simulink model "ARS308_RX"  (R2018b)
settings: Solver=FixedStepAuto  StartTime=0.0  StopTime=inf  FixedStep=0.005  RelTol=1e-3
PostLoadFcn:
  | if any(exist('dsrtsu_mdlpostloadfcn', 'file') ~= 0), dsrtsu_mdlpostloadfcn('Execute', bdroot); end
libraries: rtican x18
(part 4 of 4)

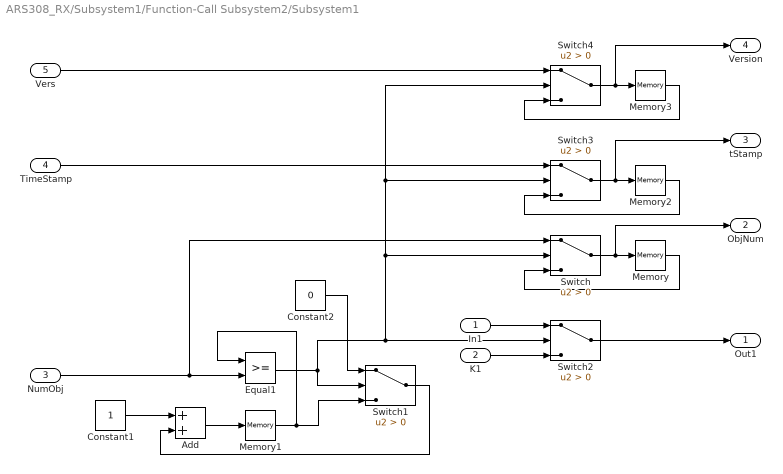
== system ARS308_RX/Subsystem1/Function-Call Subsystem2/Subsystem1 ==
  In1 : Inport
  K1 : Inport  Port=2
  NumObj : Inport  Port=3
  TimeStamp : Inport  Port=4
  Vers : Inport  Port=5
  Add : Sum
  Constant1 : Constant  OutDataTypeStr=single
  Constant2 : Constant  Value=0  OutDataTypeStr=single
  Equal1 : RelationalOperator  OutDataTypeStr=boolean  RndMeth=Simplest
  Memory : Memory  InheritSampleTime=on
  Memory1 : Memory  InitialCondition=1  InheritSampleTime=on
  Memory2 : Memory  InheritSampleTime=on
  Memory3 : Memory  InheritSampleTime=on
  Switch{,1..4} (5 alike) : Switch  Criteria=u2 > Threshold
  Out1 : Outport
  ObjNum : Outport  Port=2
  tStamp : Outport  Port=3
  Version : Outport  Port=4
  wires:
  Constant1/1 -> Add/1
  NumObj/1 -> Switch/1, Equal1/2
  K1/1 -> Switch2/3
  Constant2/1 -> Switch1/1
  Switch2/1 -> Out1/1
  Add/1 -> Memory1/1
  In1/1 -> Switch2/1
  Switch/1 -> ObjNum/1, Memory/1
  Memory/1 -> Switch/3
  Memory1/1 -> Equal1/1, Switch1/3
  Switch1/1 -> Add/2
  TimeStamp/1 -> Switch3/1
  Switch3/1 -> tStamp/1, Memory2/1
  Memory2/1 -> Switch3/3
  Equal1/1 -> Switch4/2, Switch3/2, Switch/2, Switch2/2, Switch1/2
  Memory3/1 -> Switch4/3
  Switch4/1 -> Version/1, Memory3/1
  Vers/1 -> Switch4/1

== system ARS308_RX/RTI Data/RTI Data Store/RTI Data Store/RTI Data Store ==
  RTI Data Store : Subsystem  mask(RTI_DATA_STORE){}
      mask help:
      | RTI Data Store Block. This block is used by RTI to store internal model dependent data. Deleting this block will result in data loss.
      |
      | NEVER DELETE, COPY, OR MODIFY THIS BLOCK!
      mask Help:
      | RTI Data Store Block. This block is used by RTI to store internal model dependent data. Deleting this block will result in data loss.
      | 
      | NEVER DELETE, COPY, OR MODIFY THIS BLOCK!
      mask Display: text(0.5, 0.5, ' ', 'HorizontalAlignment', 'center');

== system ARS308_RX/RTI Data/RTI Data Store/RTI Data Store/RTI Data Store/RTI Data Store ==
